simulink model "vehicle_dynamics_system"  (R2012b)
settings: Solver=ode3  StartTime=0.0  StopTime=10.0  FixedStep=T  RelTol=1e-3
PreLoadFcn:
  | init_parameters;
undefined symbols (not defined in the file): CarBody, Differential, Engine, Gearbox, Ground, Suspension, Wheel
libraries: vehicle_dynamics_lib x11, simulink x1
(part 3 of 3)

== matlab function vehicle_dynamics_system/Chassis/Wheel contact point & wheel body velocity calculation ==
  data: states input; cpFL output; rFLWheelMountPoint parameter; rFRWheelMountPoint parameter; rRLWheelMountPoint parameter; rRRWheelMountPoint parameter; cpFL1dot output; cpFR output; cpFR1dot output; cpRL output; cpRL1dot output; cpRR output; cpRR1dot output; r_DFL input; r_DFR input; r_DRL input; r_DRR input; whlFL1dot output; whlFR1dot output; whlRL1dot output; whlRR1dot output; axleFL output; axleFR output; axleRL output; axleRR output; N_GndFL input; N_GndFR input; N_GndRL input; N_GndRR input
function  [cpFL, cpFL1dot, cpFR, cpFR1dot, cpRL, cpRL1dot, cpRR, cpRR1dot, ...
    whlFL1dot, whlFR1dot, whlRL1dot, whlRR1dot, axleFL, axleFR, axleRL, axleRR] ...
    = whlcontact(states, rFLWheelMountPoint, ...
    rFRWheelMountPoint, rRLWheelMountPoint, rRRWheelMountPoint, r_DFL, r_DFR, r_DRL, r_DRR, ...
    N_GndFL,N_GndFR,N_GndRL,N_GndRR)

x_zs = states(1);
y_zs = states(2);
z_zs = states(3);
psi_zs = states(4);
theta_zs = states(5);
phi_zs = states(6);
deltaFL = states(7);
deltaFR = states(8);
zFL_zs = states(9);
zFR_zs = states(10);
zRL_zs = states(11);
zRR_zs = states(12);
% epsFL_zs = q(13);
% epsFR_zs = q(14);
% epsRL_zs = q(15);
% epsRR_zs = q(16);

x_zs1dot = states(13);
y_zs1dot = states(14);
z_zs1dot = states(15);
psi_zs1dot = states(16);
theta_zs1dot = states(17);
phi_zs1dot = states(18);
zFL_zs1dot = states(19);
zFR_zs1dot = states(20);
zRL_zs1dot = states(21);
zRR_zs1dot = states(22);
epsFL_zs1dot = states(23);
epsFR_zs1dot = states(24);
epsRL_zs1dot = states(25);
epsRR_zs1dot = states(26);


r_wheelMntFL_X = rFLWheelMountPoint(1);
r_wheelMntFL_Y = rFLWheelMountPoint(2);
r_wheelMntFL_Z = rFLWheelMountPoint(3);

r_wheelMntFR_X = rFRWheelMountPoint(1);
r_wheelMntFR_Y = rFRWheelMountPoint(2);
r_wheelMntFR_Z = rFRWheelMountPoint(3);

r_wheelMntRL_X = rRLWheelMountPoint(1);
r_wheelMntRL_Y = rRLWheelMountPoint(2);
r_wheelMntRL_Z = rRLWheelMountPoint(3);

r_wheelMntRR_X = rRRWheelMountPoint(1);
r_wheelMntRR_Y = rRRWheelMountPoint(2);
r_wheelMntRR_Z = rRRWheelMountPoint(3);

n_gndFL_X = N_GndFL(1);
n_gndFL_Y = N_GndFL(2);
n_gndFL_Z = N_GndFL(3);

n_gndFR_X = N_GndFR(1);
n_gndFR_Y = N_GndFR(2);
n_gndFR_Z = N_GndFR(3);

n_gndRL_X = N_GndRL(1);
n_gndRL_Y = N_GndRL(2);
n_gndRL_Z = N_GndRL(3);

n_gndRR_X = N_GndRR(1);
n_gndRR_Y = N_GndRR(2);
n_gndRR_Z = N_GndRR(3);


cp = zeros(12,4);

t1 = r_DFL * n_gndFL_X;
t2 = sin(psi_zs);
t3 = zFL_zs * t2;
t4 = sin(phi_zs);
t6 = cos(psi_zs);
t7 = zFL_zs * t6;
t8 = sin(theta_zs);
t9 = cos(phi_zs);
t10 = t8 * t9;
t12 = cos(theta_zs);
t13 = t6 * t12;
t15 = r_wheelMntFL_Y * t2;
t17 = r_wheelMntFL_Y * t6;
t18 = t8 * t4;
t20 = r_wheelMntFL_Z * t2;
t22 = r_wheelMntFL_Z * t6;
t25 = psi_zs1dot * t4;
t26 = t7 * t25;
t27 = zFL_zs1dot * t6;
t28 = t27 * t10;
t29 = r_DFL * n_gndFL_Z;
t31 = sin(deltaFL);
t33 = t12 * t31 * epsFL_zs1dot;
t35 = cos(deltaFL);
t36 = t29 * t35;
t37 = t2 * t8;
t38 = t4 * epsFL_zs1dot;
t39 = t37 * t38;
t41 = t2 * psi_zs1dot;
t42 = t12 * r_wheelMntFL_X;
t43 = t41 * t42;
t44 = t6 * t8;
t45 = theta_zs1dot * r_wheelMntFL_X;
t46 = t44 * t45;
t47 = psi_zs1dot * t9;
t48 = t17 * t47;
t49 = t4 * phi_zs1dot;
t50 = t15 * t49;
t51 = t9 * phi_zs1dot;
t52 = t3 * t51;
t53 = t20 * t51;
t54 = r_DFL * n_gndFL_Y;
t55 = t8 * phi_zs1dot;
t57 = t22 * t25;
t58 = t12 * theta_zs1dot;
t59 = t58 * t9;
t60 = t7 * t59;
t61 = psi_zs1dot * t8;
t62 = t61 * t9;
t63 = t3 * t62;
t64 = t26 + t28 - t29 * t2 * t33 - t36 * t39 - t43 - t46 - t48 + t50 + t52 + t53 - t54 * t55 + t57 + t60 - t63;
t65 = t18 * phi_zs1dot;
t66 = t7 * t65;
t67 = t58 * t4;
t68 = t17 * t67;
t69 = t61 * t4;
t70 = t15 * t69;
t71 = t10 * phi_zs1dot;
t72 = t17 * t71;
t73 = t20 * t62;
t74 = t22 * t59;
t75 = t22 * t65;
t78 = t35 * t4 * epsFL_zs1dot;
t80 = t31 * t8;
t81 = t80 * epsFL_zs1dot;
t83 = t6 * t9;
t84 = t83 * epsFL_zs1dot;
t86 = t6 * theta_zs1dot;
t88 = t2 * t12;
t89 = t88 * phi_zs1dot;
t91 = zFL_zs1dot * t2;
t92 = t91 * t4;
t94 = -t66 + t68 - t70 + t72 - t73 + t74 - t75 + t54 * t12 * t78 - t54 * t81 - t36 * t84 - t29 * t86 - t29 * t89 + x_zs1dot + t92 + t54 * psi_zs1dot;
t96 = t92 + t26 + t52 + t28 - t63 + t60 - t66 - t43 - t46 - t48 + t50 - t70 + t68 + t72 + t57 + t53 - t73 + t74 - t75 + x_zs1dot;
t98 = t35 * t2;
t100 = t35 * t6;
t111 = t27 * t4;
t113 = t3 * t25;
t114 = t7 * t51;
t115 = t91 * t10;
t116 = t37 * t45;
t117 = t15 * t47;
t118 = t17 * t49;
t119 = t6 * psi_zs1dot;
t120 = t119 * t42;
t121 = t7 * t62;
t122 = t3 * t59;
t123 = t3 * t65;
t124 = t20 * t25;
t125 = t2 * theta_zs1dot;
t127 = -t111 - t1 * psi_zs1dot + t113 - t114 + t115 - t116 - t117 - t118 + t120 + t121 + t122 - t123 + t124 - t29 * t125;
t129 = t22 * t51;
t130 = t22 * t62;
t131 = t20 * t65;
t132 = t20 * t59;
t133 = t15 * t67;
t134 = t17 * t69;
t135 = t15 * t71;
t139 = t44 * t38;
t143 = t13 * phi_zs1dot;
t145 = t2 * t9;
t146 = t145 * epsFL_zs1dot;
t148 = t1 * t55 - t129 + t130 - t131 + t132 + t133 + t134 + t135 - t1 * t12 * t78 + t1 * t81 + t36 * t139 + y_zs1dot + t29 * t6 * t33 + t29 * t143 - t36 * t146;
t150 = -t111 + t113 - t114 + t115 + t121 + t122 - t123 + t120 - t116 - t117 - t118 + t134 + t133 + t135 + t124 - t129 + t130 + t132 - t131 + y_zs1dot;
t155 = t12 * t9;
t158 = t12 * t4;
t162 = t58 * r_wheelMntFL_X;
t163 = t155 * zFL_zs1dot;
t165 = t155 * phi_zs1dot * r_wheelMntFL_Y;
t166 = t8 * theta_zs1dot;
t168 = t166 * t9 * zFL_zs;
t170 = t158 * phi_zs1dot * zFL_zs;
t172 = t166 * t4 * r_wheelMntFL_Y;
t174 = t166 * t9 * r_wheelMntFL_Z;
t176 = t158 * phi_zs1dot * r_wheelMntFL_Z;
t181 = t1 * t35;
t186 = t54 * t35;
t191 = -t162 + t163 + t165 - t168 - t170 - t172 - t174 - t176 - t54 * t143 + t54 * t125 + t1 * t89 + t1 * t86 + z_zs1dot + t181 * t84 + t1 * t2 * t33 + t181 * t39 - t186 * t139 - t54 * t6 * t33 + t186 * t146;
t196 = r_DFR * n_gndFR_X;
t197 = zFR_zs * t2;
t199 = zFR_zs * t6;
t202 = r_wheelMntFR_Y * t2;
t204 = r_wheelMntFR_Y * t6;
t206 = r_wheelMntFR_Z * t2;
t208 = r_wheelMntFR_Z * t6;
t211 = r_DFR * n_gndFR_Y;
t212 = sin(deltaFR);
t213 = t212 * t8;
t214 = t213 * epsFR_zs1dot;
t216 = r_DFR * n_gndFR_Z;
t217 = cos(deltaFR);
t218 = t216 * t217;
t219 = t4 * epsFR_zs1dot;
t220 = t37 * t219;
t224 = t12 * t212 * epsFR_zs1dot;
t226 = t83 * epsFR_zs1dot;
t230 = t217 * t4 * epsFR_zs1dot;
t233 = zFR_zs1dot * t2;
t234 = t233 * t4;
t237 = t197 * t51;
t238 = zFR_zs1dot * t6;
t239 = t238 * t10;
t241 = t197 * t62;
t242 = -t211 * t214 - t218 * t220 - t216 * t2 * t224 - t218 * t226 + t211 * t12 * t230 + x_zs1dot + t211 * psi_zs1dot + t234 - t211 * t55 - t216 * t86 + t237 + t239 - t216 * t89 - t241;
t243 = t199 * t59;
t244 = t199 * t65;
t245 = t202 * t69;
t246 = t204 * t71;
t247 = t204 * t67;
t248 = t12 * r_wheelMntFR_X;
t249 = t41 * t248;
t250 = theta_zs1dot * r_wheelMntFR_X;
t251 = t44 * t250;
t252 = t204 * t47;
t253 = t202 * t49;
t254 = t199 * t25;
t255 = t208 * t25;
t256 = t206 * t51;
t257 = t206 * t62;
t258 = t208 * t59;
t259 = t208 * t65;
t260 = t243 - t244 - t245 + t246 + t247 - t249 - t251 - t252 + t253 + t254 + t255 + t256 - t257 + t258 - t259;
t262 = t234 + t254 + t237 + t239 - t241 + t243 - t244 - t249 - t251 - t252 + t253 - t245 + t247 + t246 + t255 + t256 - t257 + t258 - t259 + x_zs1dot;
t264 = t217 * t2;
t266 = t217 * t6;
t277 = t197 * t25;
t278 = t199 * t51;
t279 = t119 * t248;
t280 = t37 * t250;
t281 = t233 * t10;
t282 = t202 * t67;
t283 = t204 * t69;
t284 = t202 * t71;
t285 = t208 * t62;
t286 = t206 * t65;
t287 = t206 * t59;
t288 = t197 * t59;
t289 = t199 * t62;
t290 = t197 * t65;
t291 = t277 - t278 + t279 - t280 + t281 + t282 + t283 + t284 + t285 - t286 + t287 + t288 + t289 - t290;
t292 = t202 * t47;
t293 = t204 * t49;
t294 = t206 * t25;
t295 = t208 * t51;
t298 = t44 * t219;
t300 = t145 * epsFR_zs1dot;
t309 = t238 * t4;
t310 = -t292 - t293 + t294 - t295 + t196 * t55 - t216 * t125 + t218 * t298 - t218 * t300 + t216 * t6 * t224 + t196 * t214 - t196 * t12 * t230 + t216 * t143 - t196 * psi_zs1dot - t309 + y_zs1dot;
t312 = -t309 + t277 - t278 + t281 + t289 + t288 - t290 + t279 - t280 - t292 - t293 + t283 + t282 + t284 + t294 - t295 + t285 + t287 - t286 + y_zs1dot;
t322 = t58 * r_wheelMntFR_X;
t323 = t155 * zFR_zs1dot;
t325 = t155 * phi_zs1dot * r_wheelMntFR_Y;
t328 = t166 * t9 * r_wheelMntFR_Z;
t330 = t158 * phi_zs1dot * r_wheelMntFR_Z;
t332 = t158 * phi_zs1dot * zFR_zs;
t334 = t166 * t4 * r_wheelMntFR_Y;
t336 = t166 * t9 * zFR_zs;
t337 = t196 * t217;
t344 = t211 * t217;
t350 = -t322 + t323 + t325 - t211 * t143 - t328 - t330 - t332 - t334 - t336 + z_zs1dot + t337 * t220 + t337 * t226 + t196 * t2 * t224 - t211 * t6 * t224 + t344 * t300 - t344 * t298 + t196 * t89 + t196 * t86 + t211 * t125;
t355 = r_DRL * n_gndRL_X;
t356 = zRL_zs * t2;
t358 = zRL_zs * t6;
t361 = r_wheelMntRL_Y * t2;
t363 = r_wheelMntRL_Y * t6;
t365 = r_wheelMntRL_Z * t2;
t367 = r_wheelMntRL_Z * t6;
t370 = r_DRL * n_gndRL_Z;
t371 = t83 * epsRL_zs1dot;
t374 = t18 * epsRL_zs1dot;
t376 = r_DRL * n_gndRL_Y;
t377 = t158 * epsRL_zs1dot;
t380 = zRL_zs1dot * t2;
t381 = t380 * t4;
t382 = t358 * t25;
t383 = t356 * t51;
t384 = zRL_zs1dot * t6;
t385 = t384 * t10;
t386 = t365 * t62;
t387 = t367 * t59;
t388 = t367 * t65;
t389 = t356 * t62;
t390 = -t370 * t371 - t370 * t2 * t374 + t376 * t377 + x_zs1dot + t376 * psi_zs1dot + t381 + t382 + t383 + t385 - t386 + t387 - t388 - t389;
t391 = t358 * t59;
t392 = t358 * t65;
t393 = t363 * t67;
t394 = t361 * t69;
t395 = t363 * t71;
t396 = theta_zs1dot * r_wheelMntRL_X;
t397 = t44 * t396;
t398 = t363 * t47;
t399 = t361 * t49;
t400 = t367 * t25;
t401 = t365 * t51;
t402 = t12 * r_wheelMntRL_X;
t403 = t41 * t402;
t407 = t391 - t392 + t393 - t394 + t395 - t397 - t398 + t399 + t400 + t401 - t403 - t370 * t86 - t376 * t55 - t370 * t89;
t409 = t381 + t382 + t383 + t385 - t389 + t391 - t392 - t403 - t397 - t398 + t399 - t394 + t393 + t395 + t400 + t401 - t386 + t387 - t388 + x_zs1dot;
t411 = -t145 + t44 * t4;
t423 = t384 * t4;
t424 = t367 * t62;
t425 = t365 * t59;
t427 = t365 * t65;
t428 = t365 * t25;
t429 = t367 * t51;
t430 = t358 * t51;
t431 = t380 * t10;
t432 = t119 * t402;
t433 = -t370 * t125 + t355 * t55 + t370 * t143 - t423 + t424 + t425 - t355 * psi_zs1dot - t427 + t428 - t429 - t430 + t431 + t432;
t434 = t358 * t62;
t435 = t356 * t59;
t436 = t356 * t65;
t437 = t363 * t69;
t438 = t361 * t67;
t439 = t361 * t71;
t440 = t37 * t396;
t441 = t361 * t47;
t442 = t363 * t49;
t443 = t356 * t25;
t446 = t145 * epsRL_zs1dot;
t449 = t434 + t435 - t436 + t437 + t438 + t439 + y_zs1dot - t440 - t441 - t442 + t443 + t370 * t6 * t374 - t370 * t446 - t355 * t377;
t451 = -t423 + t443 - t430 + t431 + t434 + t435 - t436 + t432 - t440 - t441 - t442 + t437 + t438 + t439 + t428 - t429 + t424 + t425 - t427 + y_zs1dot;
t453 = t83 + t37 * t4;
t464 = t155 * phi_zs1dot * r_wheelMntRL_Y;
t466 = t166 * t9 * zRL_zs;
t468 = t158 * phi_zs1dot * zRL_zs;
t473 = t166 * t9 * r_wheelMntRL_Z;
t475 = t166 * t4 * r_wheelMntRL_Y;
t478 = t158 * phi_zs1dot * r_wheelMntRL_Z;
t481 = t155 * zRL_zs1dot;
t482 = t58 * r_wheelMntRL_X;
t483 = -t376 * t143 + t376 * t125 + t355 * t86 + t355 * t89 + t464 + z_zs1dot - t466 - t468 + t376 * t446 - t376 * t6 * t374 - t473 - t475 + t355 * t371 - t478 + t355 * t2 * t374 + t481 - t482;
t485 = r_DRR * n_gndRR_X;
t486 = zRR_zs * t2;
t488 = zRR_zs * t6;
t491 = r_wheelMntRR_Y * t2;
t493 = r_wheelMntRR_Y * t6;
t495 = r_wheelMntRR_Z * t2;
t497 = r_wheelMntRR_Z * t6;
t500 = t488 * t25;
t501 = t486 * t51;
t502 = r_DRR * n_gndRR_Y;
t504 = r_DRR * n_gndRR_Z;
t506 = t495 * t62;
t507 = t497 * t59;
t508 = t497 * t65;
t509 = t486 * t62;
t510 = t488 * t59;
t511 = t488 * t65;
t512 = t491 * t69;
t513 = t493 * t67;
t514 = t493 * t71;
t515 = t500 + t501 - t502 * t55 - t504 * t86 - t506 + t507 - t508 - t509 + t510 - t511 - t512 + t513 + t514;
t516 = zRR_zs1dot * t2;
t517 = t516 * t4;
t519 = zRR_zs1dot * t6;
t520 = t519 * t10;
t521 = theta_zs1dot * r_wheelMntRR_X;
t522 = t44 * t521;
t524 = t158 * epsRR_zs1dot;
t526 = t83 * epsRR_zs1dot;
t529 = t18 * epsRR_zs1dot;
t531 = t493 * t47;
t532 = t491 * t49;
t533 = t497 * t25;
t534 = t495 * t51;
t535 = t12 * r_wheelMntRR_X;
t536 = t41 * t535;
t537 = x_zs1dot + t517 + t502 * psi_zs1dot + t520 - t522 - t504 * t89 + t502 * t524 - t504 * t526 - t504 * t2 * t529 - t531 + t532 + t533 + t534 - t536;
t539 = t517 + t500 + t501 + t520 - t509 + t510 - t511 - t536 - t522 - t531 + t532 - t512 + t513 + t514 + t533 + t534 - t506 + t507 - t508 + x_zs1dot;
t548 = t497 * t62;
t549 = t495 * t59;
t552 = t495 * t65;
t554 = t145 * epsRR_zs1dot;
t559 = t519 * t4;
t561 = t486 * t25;
t562 = t548 + t549 + t504 * t6 * t529 - t552 - t485 * t524 - t504 * t554 + t485 * t55 - t504 * t125 + t504 * t143 - t559 - t485 * psi_zs1dot + t561 + y_zs1dot;
t563 = t488 * t51;
t564 = t516 * t10;
t565 = t495 * t25;
t566 = t497 * t51;
t567 = t493 * t69;
t568 = t491 * t67;
t569 = t491 * t71;
t570 = t488 * t62;
t571 = t486 * t59;
t572 = t486 * t65;
t573 = t119 * t535;
t574 = t37 * t521;
t575 = t491 * t47;
t576 = t493 * t49;
t577 = -t563 + t564 + t565 - t566 + t567 + t568 + t569 + t570 + t571 - t572 + t573 - t574 - t575 - t576;
t579 = -t559 + t561 - t563 + t564 + t570 + t571 - t572 + t573 - t574 - t575 - t576 + t567 + t568 + t569 + t565 - t566 + t548 + t549 - t552 + y_zs1dot;
t585 = t58 * r_wheelMntRR_X;
t586 = t155 * zRR_zs1dot;
t588 = t155 * phi_zs1dot * r_wheelMntRR_Y;
t592 = t166 * t9 * zRR_zs;
t594 = t158 * phi_zs1dot * zRR_zs;
t596 = t166 * t4 * r_wheelMntRR_Y;
t598 = t166 * t9 * r_wheelMntRR_Z;
t600 = t158 * phi_zs1dot * r_wheelMntRR_Z;
t609 = -t585 + t586 + t588 + t502 * t125 + t485 * t86 - t592 - t594 - t596 - t598 - t600 + t485 * t89 - t502 * t143 + t502 * t554 - t502 * t6 * t529 + t485 * t526 + z_zs1dot + t485 * t2 * t529;
cp(1,1) = -t1 + t3 * t4 + t7 * t10 + t13 * r_wheelMntFL_X - t15 * t9 + t17 * t18 + t20 * t4 + t22 * t10 + x_zs;
cp(1,2) = t64 + t94;
cp(1,3) = t96;
cp(1,4) = t13 * t31 - t98 * t9 + t100 * t18;
cp(2,1) = -t54 - t7 * t4 + t3 * t10 + t88 * r_wheelMntFL_X + t17 * t9 + t15 * t18 - t22 * t4 + t20 * t10 + y_zs;
cp(2,2) = t127 + t148;
cp(2,3) = t150;
cp(2,4) = t88 * t31 + t100 * t9 + t98 * t18;
cp(3,1) = -t29 + t155 * zFL_zs - t8 * r_wheelMntFL_X + t158 * r_wheelMntFL_Y + t155 * r_wheelMntFL_Z + z_zs;
cp(3,2) = t191;
cp(3,3) = -t168 - t170 + t163 - t162 - t172 + t165 - t174 - t176 + z_zs1dot;
cp(3,4) = -t80 + t12 * t35 * t4;
cp(4,1) = -t196 + t197 * t4 + t199 * t10 + t13 * r_wheelMntFR_X - t202 * t9 + t204 * t18 + t206 * t4 + t208 * t10 + x_zs;
cp(4,2) = t242 + t260;
cp(4,3) = t262;
cp(4,4) = t13 * t212 - t264 * t9 + t266 * t18;
cp(5,1) = -t211 - t199 * t4 + t197 * t10 + t88 * r_wheelMntFR_X + t204 * t9 + t202 * t18 - t208 * t4 + t206 * t10 + y_zs;
cp(5,2) = t291 + t310;
cp(5,3) = t312;
cp(5,4) = t88 * t212 + t266 * t9 + t264 * t18;
cp(6,1) = -t216 + t155 * zFR_zs - t8 * r_wheelMntFR_X + t158 * r_wheelMntFR_Y + t155 * r_wheelMntFR_Z + z_zs;
cp(6,2) = t350;
cp(6,3) = -t336 - t332 + t323 - t322 - t334 + t325 - t328 - t330 + z_zs1dot;
cp(6,4) = -t213 + t12 * t217 * t4;
cp(7,1) = -t355 + t356 * t4 + t358 * t10 + t13 * r_wheelMntRL_X - t361 * t9 + t363 * t18 + t365 * t4 + t367 * t10 + x_zs;
cp(7,2) = t390 + t407;
cp(7,3) = t409;
cp(7,4) = t411;
cp(8,1) = -t376 - t358 * t4 + t356 * t10 + t88 * r_wheelMntRL_X + t363 * t9 + t361 * t18 - t367 * t4 + t365 * t10 + y_zs;
cp(8,2) = t433 + t449;
cp(8,3) = t451;
cp(8,4) = t453;
cp(9,1) = -t370 + t155 * zRL_zs - t8 * r_wheelMntRL_X + t158 * r_wheelMntRL_Y + t155 * r_wheelMntRL_Z + z_zs;
cp(9,2) = t483;
cp(9,3) = -t466 - t468 + t481 - t482 - t475 + t464 - t473 - t478 + z_zs1dot;
cp(9,4) = t158;
cp(10,1) = -t485 + t486 * t4 + t488 * t10 + t13 * r_wheelMntRR_X - t491 * t9 + t493 * t18 + t495 * t4 + t497 * t10 + x_zs;
cp(10,2) = t515 + t537;
cp(10,3) = t539;
cp(10,4) = t411;
cp(11,1) = -t502 - t488 * t4 + t486 * t10 + t88 * r_wheelMntRR_X + t493 * t9 + t491 * t18 - t497 * t4 + t495 * t10 + y_zs;
cp(11,2) = t562 + t577;
cp(11,3) = t579;
cp(11,4) = t453;
cp(12,1) = -t504 + t155 * zRR_zs - t8 * r_wheelMntRR_X + t158 * r_wheelMntRR_Y + t155 * r_wheelMntRR_Z + z_zs;
cp(12,2) = t609;
cp(12,3) = -t592 - t594 + t586 - t585 - t596 + t588 - t598 - t600 + z_zs1dot;
cp(12,4) = t158;


cpFL = cp(1:3,1);
cpFR = cp(4:6,1);
cpRL = cp(7:9,1);
cpRR = cp(10:12,1);

cpFL1dot = cp(1:3,2);
cpFR1dot = cp(4:6,2);
cpRL1dot = cp(7:9,2);
cpRR1dot = cp(10:12,2);

whlFL1dot = cp(1:3,3);
whlFR1dot = cp(4:6,3);
whlRL1dot = cp(7:9,3);
whlRR1dot = cp(10:12,3);

axleFL = cp(1:3,4);
axleFR = cp(4:6,4);
axleRL = cp(7:9,4);
axleRR = cp(10:12,4);
